simulink model "switch_test"  (R2022b)
settings: Solver=VariableStepAuto  StartTime=0.0  StopTime=20  RelTol=1e-3
undefined symbols (not defined in the file): initmatrix
settings Model: Creator=Dong  LastModifiedBy=r.dong

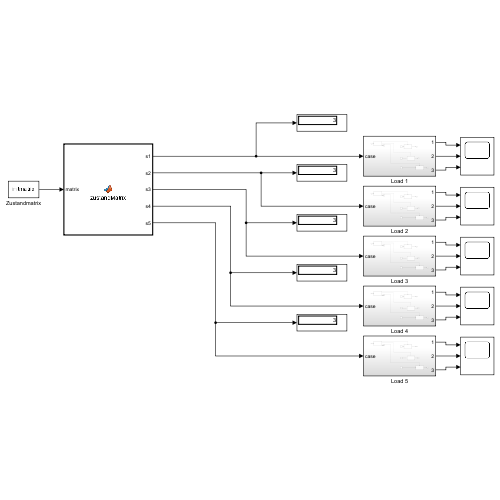
[thumbnail: Simulink's stored preview of the top-level diagram]
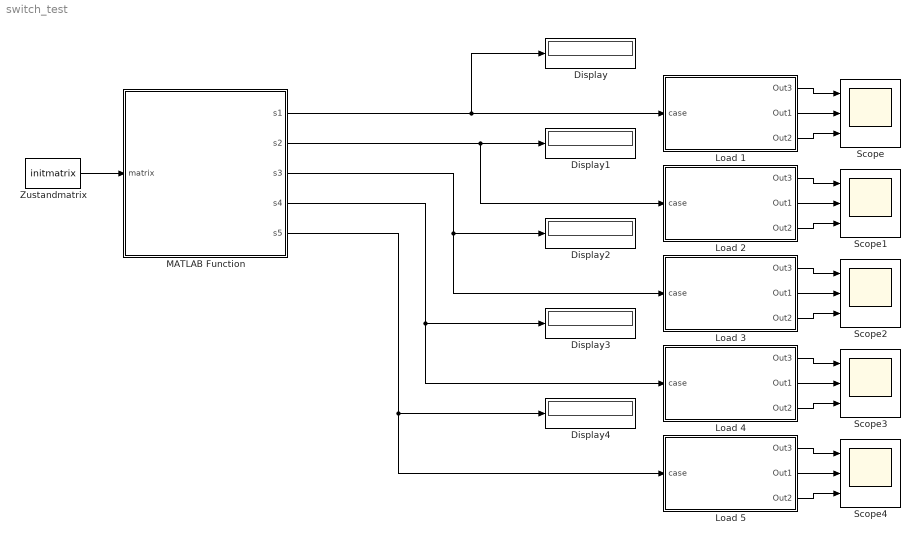
== system switch_test ==
  Display{,1..4} (5 alike) : Display
  Load 1 : Subsystem
  Load 2 : Subsystem
  Load 3 : Subsystem
  Load 4 : Subsystem
  Load 5 : Subsystem
  MATLAB Function : MATLAB Function  TreatAsAtomicUnit=on
  Scope{,1..4} (5 alike) : Scope  NumInputPorts=3
  Zustandmatrix : Constant  Value=initmatrix
  wires:
  Zustandmatrix/1 -> MATLAB Function/1(matrix)
  MATLAB Function/1(s1) -> Display/1, Load 1/1(case)
  Load 1/1(Out3) -> Scope/1
  Load 1/2(Out1) -> Scope/2
  Load 1/3(Out2) -> Scope/3
  Load 2/3(Out2) -> Scope1/3
  Load 2/2(Out1) -> Scope1/2
  Load 2/1(Out3) -> Scope1/1
  Load 4/1(Out3) -> Scope3/1
  Load 4/2(Out1) -> Scope3/2
  Load 4/3(Out2) -> Scope3/3
  Load 3/3(Out2) -> Scope2/3
  Load 3/2(Out1) -> Scope2/2
  Load 3/1(Out3) -> Scope2/1
  Load 5/3(Out2) -> Scope4/3
  Load 5/2(Out1) -> Scope4/2
  Load 5/1(Out3) -> Scope4/1
  MATLAB Function/2(s2) -> Load 2/1(case), Display1/1
  MATLAB Function/3(s3) -> Display2/1, Load 3/1(case)
  MATLAB Function/4(s4) -> Display3/1, Load 4/1(case)
  MATLAB Function/5(s5) -> Load 5/1(case), Display4/1

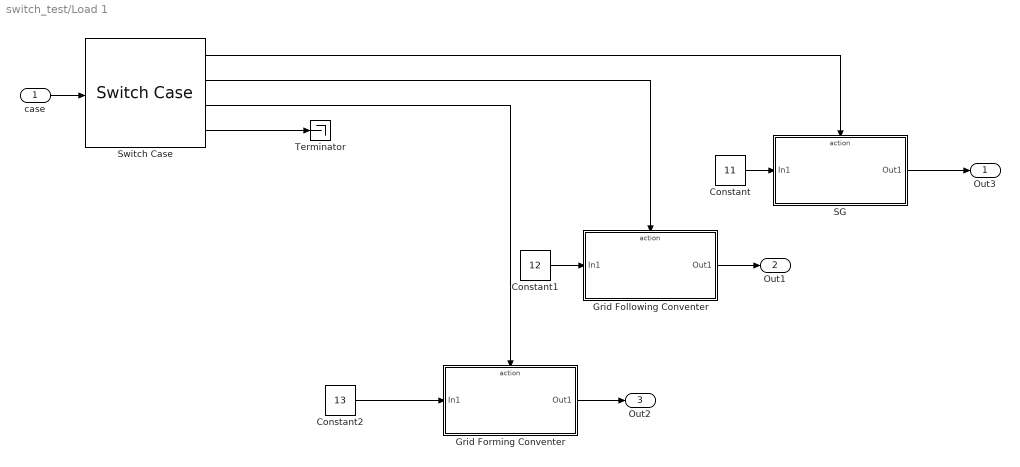
== system switch_test/Load 1 ==
  case : Inport
  Constant : Constant  Value=11
  Constant1 : Constant  Value=12
  Constant2 : Constant  Value=13
  Grid Following Conventer : Subsystem  TreatAsAtomicUnit=on
  Grid Forming Conventer : Subsystem  TreatAsAtomicUnit=on
  SG : Subsystem  TreatAsAtomicUnit=on
  Switch Case : SwitchCase  CaseConditions={1,[2],[3]}
  Terminator : Terminator
  Out3 : Outport
  Out1 : Outport  Port=2
  Out2 : Outport  Port=3
  wires:
  case/1 -> Switch Case/1
  Switch Case/1 -> SG/Action
  Switch Case/3 -> Grid Forming Conventer/Action
  Switch Case/4 -> Terminator/1
  SG/1(Out1) -> Out3/1
  Switch Case/2 -> Grid Following Conventer/Action
  Constant/1 -> SG/1(In1)
  Constant1/1 -> Grid Following Conventer/1(In1)
  Constant2/1 -> Grid Forming Conventer/1(In1)
  Grid Following Conventer/1(Out1) -> Out1/1
  Grid Forming Conventer/1(Out1) -> Out2/1

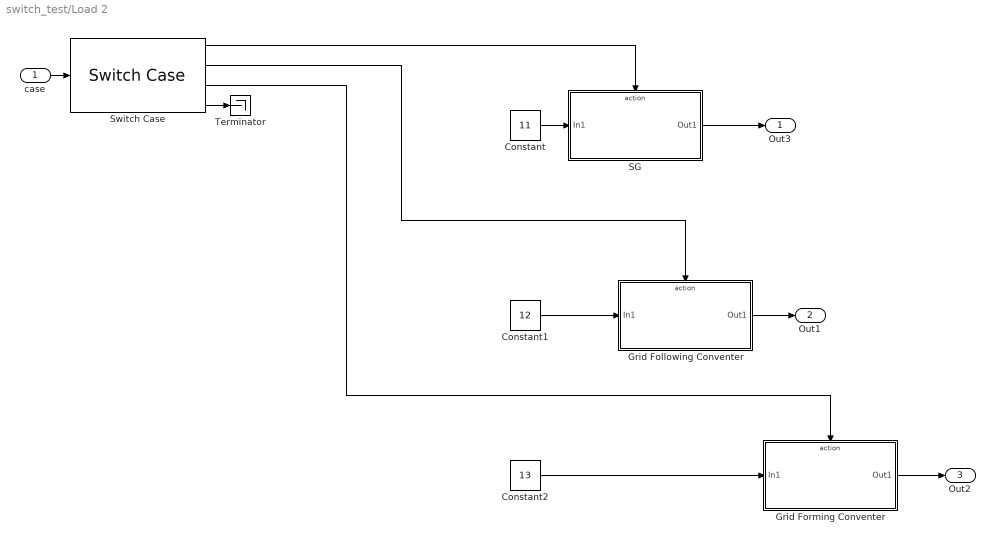
== system switch_test/Load 2 ==
  case : Inport
  Constant : Constant  Value=11
  Constant1 : Constant  Value=12
  Constant2 : Constant  Value=13
  Grid Following Conventer : Subsystem  TreatAsAtomicUnit=on
  Grid Forming Conventer : Subsystem  TreatAsAtomicUnit=on
  SG : Subsystem  TreatAsAtomicUnit=on
  Switch Case : SwitchCase  CaseConditions={1,[2],[3]}
  Terminator : Terminator
  Out3 : Outport
  Out1 : Outport  Port=2
  Out2 : Outport  Port=3
  wires:
  Grid Forming Conventer/1(Out1) -> Out2/1
  Grid Following Conventer/1(Out1) -> Out1/1
  Constant2/1 -> Grid Forming Conventer/1(In1)
  Constant1/1 -> Grid Following Conventer/1(In1)
  Constant/1 -> SG/1(In1)
  Switch Case/2 -> Grid Following Conventer/Action
  SG/1(Out1) -> Out3/1
  Switch Case/4 -> Terminator/1
  Switch Case/3 -> Grid Forming Conventer/Action
  Switch Case/1 -> SG/Action
  case/1 -> Switch Case/1

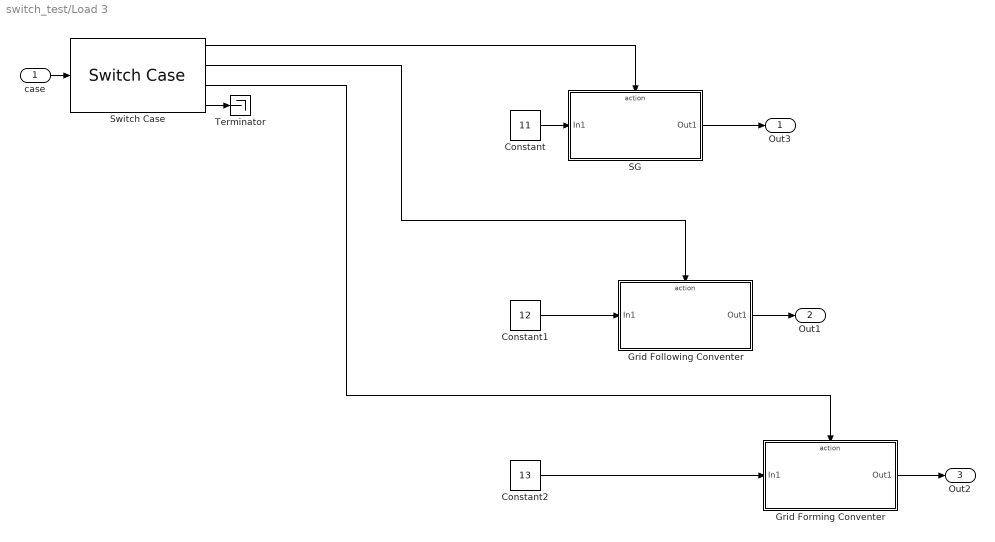
== system switch_test/Load 3 ==
  case : Inport
  Constant : Constant  Value=11
  Constant1 : Constant  Value=12
  Constant2 : Constant  Value=13
  Grid Following Conventer : Subsystem  TreatAsAtomicUnit=on
  Grid Forming Conventer : Subsystem  TreatAsAtomicUnit=on
  SG : Subsystem  TreatAsAtomicUnit=on
  Switch Case : SwitchCase  CaseConditions={1,[2],[3]}
  Terminator : Terminator
  Out3 : Outport
  Out1 : Outport  Port=2
  Out2 : Outport  Port=3
  wires:
  case/1 -> Switch Case/1
  Switch Case/1 -> SG/Action
  Switch Case/3 -> Grid Forming Conventer/Action
  Switch Case/4 -> Terminator/1
  SG/1(Out1) -> Out3/1
  Switch Case/2 -> Grid Following Conventer/Action
  Constant/1 -> SG/1(In1)
  Constant1/1 -> Grid Following Conventer/1(In1)
  Constant2/1 -> Grid Forming Conventer/1(In1)
  Grid Following Conventer/1(Out1) -> Out1/1
  Grid Forming Conventer/1(Out1) -> Out2/1

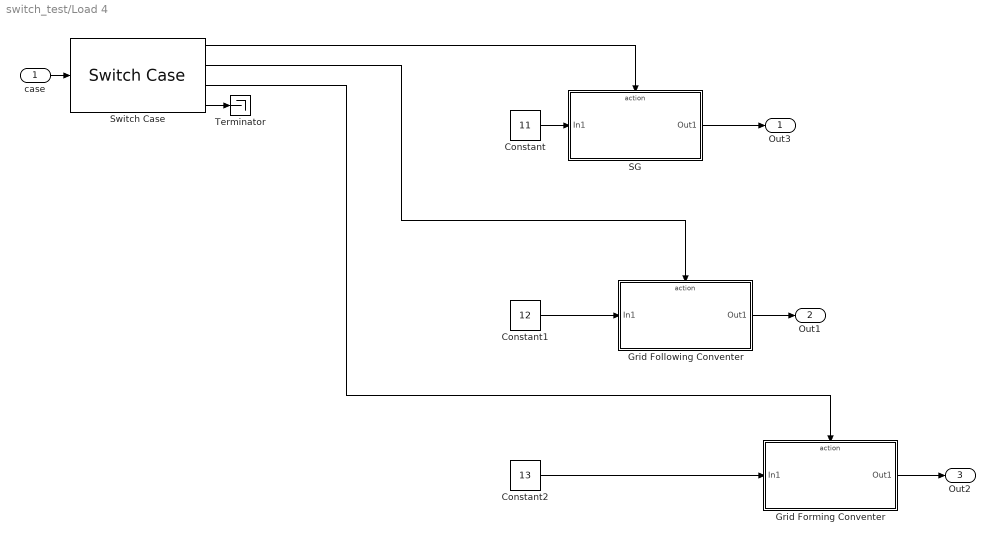
== system switch_test/Load 4 ==
  case : Inport
  Constant : Constant  Value=11
  Constant1 : Constant  Value=12
  Constant2 : Constant  Value=13
  Grid Following Conventer : Subsystem  TreatAsAtomicUnit=on
  Grid Forming Conventer : Subsystem  TreatAsAtomicUnit=on
  SG : Subsystem  TreatAsAtomicUnit=on
  Switch Case : SwitchCase  CaseConditions={1,[2],[3]}
  Terminator : Terminator
  Out3 : Outport
  Out1 : Outport  Port=2
  Out2 : Outport  Port=3
  wires:
  Grid Forming Conventer/1(Out1) -> Out2/1
  Grid Following Conventer/1(Out1) -> Out1/1
  Constant2/1 -> Grid Forming Conventer/1(In1)
  Constant1/1 -> Grid Following Conventer/1(In1)
  Constant/1 -> SG/1(In1)
  Switch Case/2 -> Grid Following Conventer/Action
  SG/1(Out1) -> Out3/1
  Switch Case/4 -> Terminator/1
  Switch Case/3 -> Grid Forming Conventer/Action
  Switch Case/1 -> SG/Action
  case/1 -> Switch Case/1

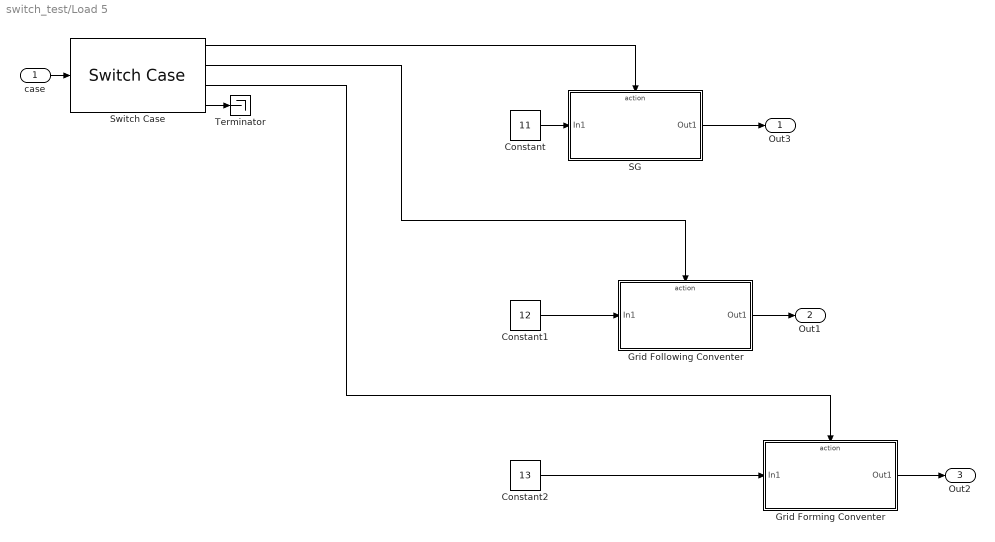
== system switch_test/Load 5 ==
  case : Inport
  Constant : Constant  Value=11
  Constant1 : Constant  Value=12
  Constant2 : Constant  Value=13
  Grid Following Conventer : Subsystem  TreatAsAtomicUnit=on
  Grid Forming Conventer : Subsystem  TreatAsAtomicUnit=on
  SG : Subsystem  TreatAsAtomicUnit=on
  Switch Case : SwitchCase  CaseConditions={1,[2],[3]}
  Terminator : Terminator
  Out3 : Outport
  Out1 : Outport  Port=2
  Out2 : Outport  Port=3
  wires:
  case/1 -> Switch Case/1
  Switch Case/1 -> SG/Action
  Switch Case/3 -> Grid Forming Conventer/Action
  Switch Case/4 -> Terminator/1
  SG/1(Out1) -> Out3/1
  Switch Case/2 -> Grid Following Conventer/Action
  Constant/1 -> SG/1(In1)
  Constant1/1 -> Grid Following Conventer/1(In1)
  Constant2/1 -> Grid Forming Conventer/1(In1)
  Grid Following Conventer/1(Out1) -> Out1/1
  Grid Forming Conventer/1(Out1) -> Out2/1

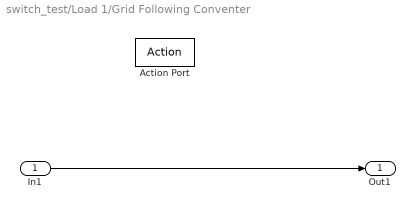
== system switch_test/Load 1/Grid Following Conventer ==
  In1 : Inport
  Action Port : ActionPort  ActionPortLabel=case [ 2 ]:
  Out1 : Outport
  wires:
  In1/1 -> Out1/1

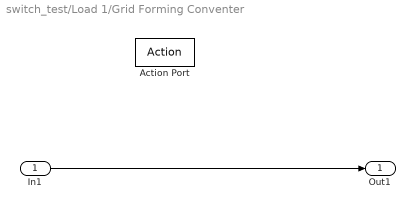
== system switch_test/Load 1/Grid Forming Conventer ==
  In1 : Inport
  Action Port : ActionPort  ActionPortLabel=case [ 3 ]:
  Out1 : Outport
  wires:
  In1/1 -> Out1/1

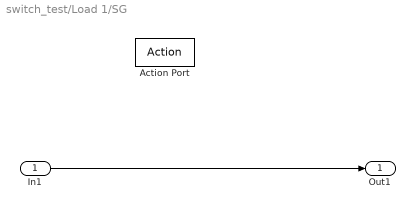
== system switch_test/Load 1/SG ==
  In1 : Inport
  Action Port : ActionPort  ActionPortLabel=case [ 1 ]:
  Out1 : Outport
  wires:
  In1/1 -> Out1/1

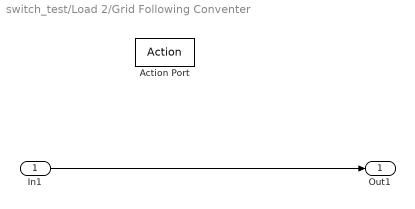
== system switch_test/Load 2/Grid Following Conventer ==
  In1 : Inport
  Action Port : ActionPort  ActionPortLabel=case [ 2 ]:
  Out1 : Outport
  wires:
  In1/1 -> Out1/1

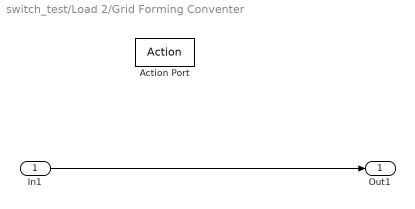
== system switch_test/Load 2/Grid Forming Conventer ==
  In1 : Inport
  Action Port : ActionPort  ActionPortLabel=case [ 3 ]:
  Out1 : Outport
  wires:
  In1/1 -> Out1/1

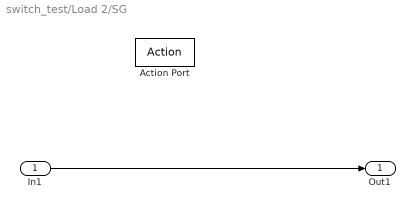
== system switch_test/Load 2/SG ==
  In1 : Inport
  Action Port : ActionPort  ActionPortLabel=case [ 1 ]:
  Out1 : Outport
  wires:
  In1/1 -> Out1/1

== system switch_test/Load 3/Grid Following Conventer ==
  In1 : Inport
  Action Port : ActionPort  ActionPortLabel=case [ 2 ]:
  Out1 : Outport
  wires:
  In1/1 -> Out1/1

== system switch_test/Load 3/Grid Forming Conventer ==
  In1 : Inport
  Action Port : ActionPort  ActionPortLabel=case [ 3 ]:
  Out1 : Outport
  wires:
  In1/1 -> Out1/1

== system switch_test/Load 3/SG ==
  In1 : Inport
  Action Port : ActionPort  ActionPortLabel=case [ 1 ]:
  Out1 : Outport
  wires:
  In1/1 -> Out1/1

== system switch_test/Load 4/Grid Following Conventer ==
  In1 : Inport
  Action Port : ActionPort  ActionPortLabel=case [ 2 ]:
  Out1 : Outport
  wires:
  In1/1 -> Out1/1

== system switch_test/Load 4/Grid Forming Conventer ==
  In1 : Inport
  Action Port : ActionPort  ActionPortLabel=case [ 3 ]:
  Out1 : Outport
  wires:
  In1/1 -> Out1/1

== system switch_test/Load 4/SG ==
  In1 : Inport
  Action Port : ActionPort  ActionPortLabel=case [ 1 ]:
  Out1 : Outport
  wires:
  In1/1 -> Out1/1

== system switch_test/Load 5/Grid Following Conventer ==
  In1 : Inport
  Action Port : ActionPort  ActionPortLabel=case [ 2 ]:
  Out1 : Outport
  wires:
  In1/1 -> Out1/1

== system switch_test/Load 5/Grid Forming Conventer ==
  In1 : Inport
  Action Port : ActionPort  ActionPortLabel=case [ 3 ]:
  Out1 : Outport
  wires:
  In1/1 -> Out1/1

== system switch_test/Load 5/SG ==
  In1 : Inport
  Action Port : ActionPort  ActionPortLabel=case [ 1 ]:
  Out1 : Outport
  wires:
  In1/1 -> Out1/1

== matlab function switch_test/MATLAB Function ==
  data: s1 output; matrix input; s2 output; s3 output; s4 output; s5 output
function [s1,s2,s3,s4,s5] = zustandMatrix(matrix)

s1 = matrix(1);
s2 = matrix(2);
s3 = matrix(3);
s4 = matrix(4);
s5 = matrix(5);
